simulink model "dinamica_fk"  (Simulink 7.5)
settings: Solver=ode3  StartTime=0.0  StopTime=19.99  FixedStep=0.01  RelTol=1e-3
settings Model: Creator=Granziera  LastModifiedBy=Granziera

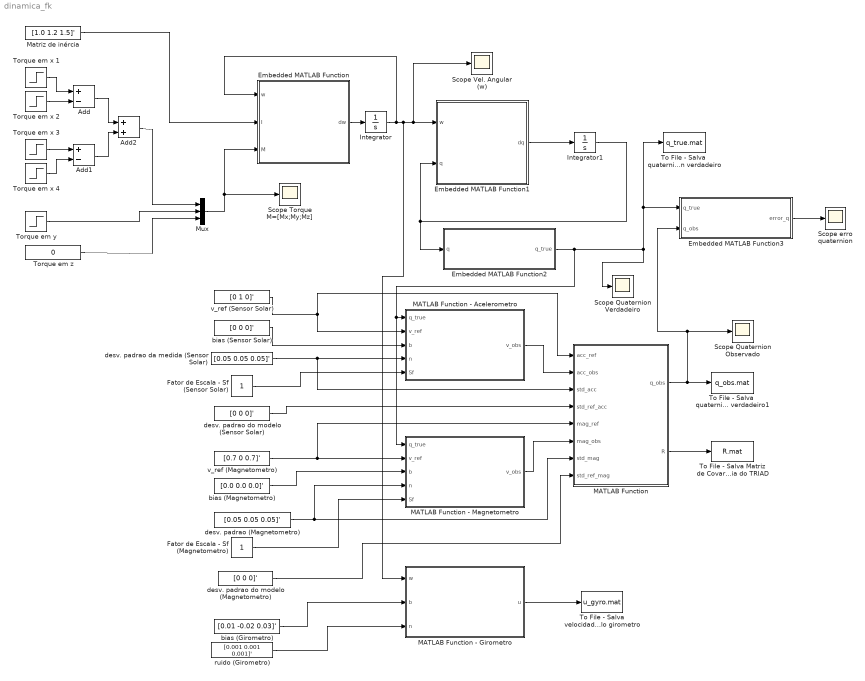
== system dinamica_fk ==
  Add : Sum  Inputs=+-
  Add1 : Sum  Inputs=+-
  Add2 : Sum
  Embedded MATLAB Function : Stateflow chart  TreatAsAtomicUnit=on
  Embedded MATLAB Function1 : Stateflow chart  TreatAsAtomicUnit=on
  Embedded MATLAB Function2 : Stateflow chart  TreatAsAtomicUnit=on
  Embedded MATLAB Function3 : Stateflow chart  TreatAsAtomicUnit=on
  Fator de Escala - Sf (Magnetometro) : Constant
  Fator de Escala - Sf (Sensor Solar) : Constant
  Integrator : Integrator  InitialCondition=[0 0 0]
  Integrator1 : Integrator  InitialCondition=[0 0 0 1]
  MATLAB Function : Stateflow chart  TreatAsAtomicUnit=on
  MATLAB Function - Acelerometro : Stateflow chart  TreatAsAtomicUnit=on
  MATLAB Function - Girometro : Stateflow chart  TreatAsAtomicUnit=on
  MATLAB Function - Magnetometro : Stateflow chart  TreatAsAtomicUnit=on
  Matriz de inércia : Constant  Value=[1.0 1.2 1.5]'
  Mux : Mux  Inputs=3
  Scope Quaternion Observado : Scope
      settings: SaveName=ScopeData3
  Scope Quaternion Verdadeiro : Scope
  Scope Torque M=[Mx;My;Mz] : Scope
      settings: YMin=-0.4  YMax=0.4  SaveName=ScopeData2
  Scope Vel. Angular (w) : Scope
  Scope erro quaternion : Scope
      settings: SaveName=ScopeData5
  To File - Salva  quaternion verdadeiro : ToFile  Filename=q_true.mat  MatrixName=q_true  SaveFormat=Timeseries
  To File - Salva  quaternion verdadeiro1 : ToFile  Filename=q_obs.mat  MatrixName=q_obs  SaveFormat=Timeseries
  To File - Salva Matriz de Covariancia do TRIAD : ToFile  Filename=R.mat  MatrixName=R  SaveFormat=Timeseries
  To File - Salva velocidade angular medida pelo girometro : ToFile  Filename=u_gyro.mat  MatrixName=u_gyro  SaveFormat=Timeseries
  Torque em x 1 : Step  Time=10  After=0.25  SampleTime=0
  Torque em x 2 : Step  Time=11  After=.25  SampleTime=0
  Torque em x 3 : Step  Time=21  After=-.25  SampleTime=0
  Torque em x 4 : Step  Time=22  After=-0.25  SampleTime=0
  "Torque em y " : Step  Time=2  Before=0.1  After=0  SampleTime=0
  Torque em z : Constant  Value=0
  bias (Girometro) : Constant  Value=[0.01 -0.02 0.03]'
  bias (Magnetometro) : Constant  Value=[0.0 0.0 0.0]'
  bias (Sensor Solar) : Constant  Value=[0 0 0]'
  desv. padrao (Magnetometro) : Constant  Value=[0.05 0.05 0.05]'
  desv. padrao da medida (Sensor Solar) : Constant  Value=[0.05 0.05 0.05]'
  desv. padrao do modelo (Magnetometro) : Constant  Value=[0 0 0]'
  desv. padrao do modelo (Sensor Solar) : Constant  Value=[0 0 0]'
  ruido (Girometro) : Constant  Value=[0.001 0.001 0.001]'
  v_ref (Magnetometro) : Constant  Value=[0.7 0 0.7]'
  v_ref (Sensor Solar) : Constant  Value=[0 1 0]'
  wires:
  Matriz de inércia/1 -> Embedded MATLAB Function/2(I)
  Embedded MATLAB Function/1(dw) -> Integrator/1
  Integrator/1 -> Embedded MATLAB Function/1(w), Embedded MATLAB Function1/1(w), Scope Vel. Angular (w)/1, MATLAB Function - Girometro/1(w)
  Mux/1 -> Embedded MATLAB Function/3(M), Scope Torque M=[Mx;My;Mz]/1
  Embedded MATLAB Function1/1(dq) -> Integrator1/1
  Integrator1/1 -> Embedded MATLAB Function1/2(q), Embedded MATLAB Function2/1(q)
  "Torque em y "/1 -> Mux/2
  Torque em z/1 -> Mux/3
  v_ref (Sensor Solar)/1 -> MATLAB Function - Acelerometro/2(v_ref), MATLAB Function/1(acc_ref)
  bias (Sensor Solar)/1 -> MATLAB Function - Acelerometro/3(b)
  desv. padrao da medida (Sensor Solar)/1 -> MATLAB Function - Acelerometro/4(n), MATLAB Function/3(std_acc)
  v_ref (Magnetometro)/1 -> MATLAB Function - Magnetometro/2(v_ref), MATLAB Function/5(mag_ref)
  bias (Magnetometro)/1 -> MATLAB Function - Magnetometro/3(b)
  bias (Girometro)/1 -> MATLAB Function - Girometro/2(b)
  ruido (Girometro)/1 -> MATLAB Function - Girometro/3(n)
  MATLAB Function - Magnetometro/1(v_obs) -> MATLAB Function/6(mag_obs)
  MATLAB Function/2(R) -> To File - Salva Matriz de Covariancia do TRIAD/1
  MATLAB Function - Girometro/1(u) -> To File - Salva velocidade angular medida pelo girometro/1
  desv. padrao (Magnetometro)/1 -> MATLAB Function - Magnetometro/4(n), MATLAB Function/7(std_mag)
  Fator de Escala - Sf (Magnetometro)/1 -> MATLAB Function - Magnetometro/5(Sf)
  Fator de Escala - Sf (Sensor Solar)/1 -> MATLAB Function - Acelerometro/5(Sf)
  desv. padrao do modelo (Sensor Solar)/1 -> MATLAB Function/4(std_ref_acc)
  MATLAB Function/1(q_obs) -> To File - Salva  quaternion verdadeiro1/1, Scope Quaternion Observado/1, Embedded MATLAB Function3/2(q_obs)
  desv. padrao do modelo (Magnetometro)/1 -> MATLAB Function/8(std_ref_mag)
  MATLAB Function - Acelerometro/1(v_obs) -> MATLAB Function/2(acc_obs)
  Embedded MATLAB Function2/1(q_true) -> Scope Quaternion Verdadeiro/1, Embedded MATLAB Function3/1(q_true), To File - Salva  quaternion verdadeiro/1, MATLAB Function - Magnetometro/1(q_true), MATLAB Function - Acelerometro/1(q_true)
  Embedded MATLAB Function3/1(error_q) -> Scope erro quaternion/1
  Torque em x 1/1 -> Add/1
  Torque em x 2/1 -> Add/2
  Torque em x 3/1 -> Add1/1
  Torque em x 4/1 -> Add1/2
  Add1/1 -> Add2/2
  Add/1 -> Add2/1
  Add2/1 -> Mux/1

== matlab function Embedded MATLAB Function1 ==
  data: w input double; dq output double; q input double
function dq = eq_cinematica(w,q)

wx = w(1);
wy = w(2);
wz = w(3);

W = [ 0    wz  -wy  wx;
     -wz   0    wx  wy;
      wy  -wx   0   wz;
     -wx  -wy  -wz  0];

dq = 1/2 * W * q;

== matlab function Embedded MATLAB Function ==
  data: w input double; dw output double; I input double; M input double
function dw = eq_dinamica(w,I,M)

wx = w(1);
wy = w(2);
wz = w(3);

Ix = I(1);
Iy = I(2);
Iz = I(3);

Mx = M(1);
My = M(2);
Mz = M(3);

dx = (Mx - wy*wz*(Iz - Iy)) / Ix;
dy = (My - wx*wz*(Ix - Iz)) / Iy;
dz = (Mz - wx*wy*(Iy - Ix)) / Iz;

dw = [dx dy dz]';

== matlab function MATLAB Function - Magnetometro ==
  data: q_true input double; v_obs output double; v_ref input double; b input double; n input double; Sf input double
function v_obs = Bloco_simula_sensor(q_true,v_ref,b,n,Sf)
%#codegen


% %Operação de transformação de quaternion para Matriz de Rotação
% q2RotMat = [q_true(4).^2 + q_true(1).^2 - q_true(2).^2 - q_true(3).^2 , 2*(q_true(1)*q_true(2) - q_true(4)*q_true(3)) , 2*(q_true(1)*q_true(3) + q_true(4)*q_true(2)) ;...
%     2*(q_true(1)*q_true(2) + q_true(4)*q_true(3)) , q_true(4).^2 - q_true(1).^2 + q_true(2).^2 - q_true(3).^2 , 2*(q_true(2)*q_true(3) - q_true(4)*q_true(1)) ;...
%     2*(q_true(1)*q_true(3) - q_true(4)*q_true(2)), 2*(q_true(2)*q_true(3) + q_true(4)*q_true(1)) , q_true(4).^2 - q_true(1).^2 - q_true(2).^2 + q_true(3).^2];

%Operação de transformação de quaternion para Matriz de Rotação
q2RotMat = [q_true(4).^2 + q_true(1).^2 - q_true(2).^2 - q_true(3).^2 , 2*(q_true(1)*q_true(2) + q_true(4)*q_true(3)) , 2*(q_true(1)*q_true(3) - q_true(4)*q_true(2)) ;...
    2*(q_true(1)*q_true(2) - q_true(4)*q_true(3)) , q_true(4).^2 - q_true(1).^2 + q_true(2).^2 - q_true(3).^2 , 2*(q_true(2)*q_true(3) + q_true(4)*q_true(1)) ;...
    2*(q_true(1)*q_true(3) + q_true(4)*q_true(2)), 2*(q_true(2)*q_true(3) - q_true(4)*q_true(1)) , q_true(4).^2 - q_true(1).^2 - q_true(2).^2 + q_true(3).^2];

%Rotaciona o vetor de observação a partir do vetor de referencia
v_rot = q2RotMat * v_ref;
%Adiciona bias e aplica o fator de escala dos sensores
v_obs = Sf * v_rot + b;
%Adiciona ruido
v_obs = v_obs + n * randn;

== matlab function MATLAB Function - Acelerometro ==
  data: q_true input double; v_obs output double; v_ref input double; b input double; n input double; Sf input double
function v_obs = Bloco_simula_sensor(q_true,v_ref,b,n,Sf)
%#codegen

% %Operação de transformação de quaternion para Matriz de Rotação
% q2RotMat = [q_true(4).^2 + q_true(1).^2 - q_true(2).^2 - q_true(3).^2 , 2*(q_true(1)*q_true(2) - q_true(4)*q_true(3)) , 2*(q_true(1)*q_true(3) + q_true(4)*q_true(2)) ;...
%     2*(q_true(1)*q_true(2) + q_true(4)*q_true(3)) , q_true(4).^2 - q_true(1).^2 + q_true(2).^2 - q_true(3).^2 , 2*(q_true(2)*q_true(3) - q_true(4)*q_true(1)) ;...
%     2*(q_true(1)*q_true(3) - q_true(4)*q_true(2)), 2*(q_true(2)*q_true(3) + q_true(4)*q_true(1)) , q_true(4).^2 - q_true(1).^2 - q_true(2).^2 + q_true(3).^2];

%Operação de transformação de quaternion para Matriz de Rotação
q2RotMat = [q_true(4).^2 + q_true(1).^2 - q_true(2).^2 - q_true(3).^2 , 2*(q_true(1)*q_true(2) + q_true(4)*q_true(3)) , 2*(q_true(1)*q_true(3) - q_true(4)*q_true(2)) ;...
    2*(q_true(1)*q_true(2) - q_true(4)*q_true(3)) , q_true(4).^2 - q_true(1).^2 + q_true(2).^2 - q_true(3).^2 , 2*(q_true(2)*q_true(3) + q_true(4)*q_true(1)) ;...
    2*(q_true(1)*q_true(3) + q_true(4)*q_true(2)), 2*(q_true(2)*q_true(3) - q_true(4)*q_true(1)) , q_true(4).^2 - q_true(1).^2 - q_true(2).^2 + q_true(3).^2];

%Rotaciona o vetor de observação a partir do vetor de referencia
v_rot = q2RotMat * v_ref;
%Adiciona bias e aplica o fator de escala dos sensores
v_obs = Sf * v_rot + b;
%Adiciona ruido
v_obs = v_obs + n * randn;

== matlab function MATLAB Function - Girometro ==
  data: w input double; u output double; b input double; n input double
function u = Bloco_simula_gyro(w,b,n)
%#codegen

%Adiciona bias
u = w + b;
%Adiciona ruido
u = u + n * randn;

== matlab function MATLAB Function ==
  data: acc_ref input double; q_obs output double; acc_obs input double; std_acc input double; std_ref_acc input double; mag_ref input double; mag_obs input double; std_mag input double; R output double; std_ref_mag input double
function [q_obs,R] = TRIAD(acc_ref,acc_obs,std_acc,std_ref_acc,mag_ref,mag_obs,std_mag,std_ref_mag)
%#codegen

%define quaternion de observacao
q_obs= zeros(4,1);

V1 = acc_ref;
W1 = acc_obs;
std_W1 = std_acc';
std_V1 = std_ref_acc';

V2 = mag_ref;
W2 = mag_obs;
std_W2 = std_mag';
std_V2 = std_ref_mag';

%normalizaçao dos vetores

V1 = V1/norm(V1);
W1 = W1/norm(W1);

V2 = V2/norm(V2);
W2 = W2/norm(W2);

%algoritmo TRIAD

M_ref = [ V1 , cross(V1,V2)/norm(cross(V1,V2)) , cross(V1,(cross(V1,V2)))/norm(cross(V1,V2)) ];

M_obs = [ W1 , cross(W1,W2)/norm(cross(W1,W2)) , cross(W1,(cross(W1,W2)))/norm(cross(W1,W2)) ];

A = M_obs * M_ref';

%--------------------------------------------------------------------------
%
%Transformação da Matriz A em quatenion de observacao
%q_obs= [q4,q1,q2,q3];

q_obs(4) = 0.5 * sqrt(trace(A)+1);
q_obs(1) = (A(2,3)-A(3,2))/(4*q_obs(4));
q_obs(2) = (A(3,1)-A(1,3))/(4*q_obs(4));
q_obs(3) = (A(1,2)-A(2,1))/(4*q_obs(4));

%Normalizando o quaternion
q_obs=q_obs/norm(q_obs);

%tira a redundancia do quaternion
if (q_obs(4)<0)
    q_obs=-q_obs;
end

%--------------------------------------------------------------------------



%Calculo da matriz de covariancia

sig1 = sqrt(std_V1.^2 + std_W1.^2);
sig2 = sqrt(std_V2.^2 + std_W2.^2);

% R = sig1.^2 * eye(3) + (1/norm(cross(W1,W2)))^2 * (sig1.^2 * (W1*W2') * (W1*W2' + W2*W1')...
%     + (sig2.^2 - sig1.^2) * W1 * W1');
R = [sig1(1)^2,0,0;0,sig1(2)^2,0;0,0,sig1(3)^2] + (1/norm(cross(W1,W2)))^2 * ([sig1(1)^2,0,0;0,sig1(2)^2,0;0,0,sig1(3)^2] * (W1*W2') * (W1*W2' + W2*W1')...
    + ([sig2(1)^2,0,0;0,sig2(2)^2,0;0,0,sig2(3)^2] - [sig1(1)^2,0,0;0,sig1(2)^2,0;0,0,sig1(3)^2]) * W1 * W1');

== matlab function Embedded MATLAB Function2 ==
  data: q_true output double; q input double
function q_true = tira_redundancia(q)

if(q(4)<0)
    q=-q;
end

q_true=q;

== matlab function Embedded MATLAB Function3 ==
  data: error_q output double; q_true input double; q_obs input double
function error_q  = error_quaternion(q_true,q_obs)
%function [euler_true,euler_obs] = quat2obs(q_true,q_obs)

% %q_true --> euler_true
% psi_true = atan((2*q_true(1)*q_true(2)+2*q_true(4)*q_true(3))/(2*q_true(4)^2+2*q_true(1)^2-1));
% theta_true = asin(-2*q_true(1)*q_true(3)+2*q_true(4)*q_true(1));
% phi_true= atan((2*q_true(2)*q_true(3)+2*q_true(4)*q_true(1))/(2*q_true(4)^2+2*q_true(3)^2-1));
% 
% euler_true = [psi_true,theta_true,phi_true];
% %conversao de radiano para graus
% euler_true = euler_true * 180/pi;
% 
% %q_obs --> euler_obs
% psi_obs = atan((2*q_obs(1)*q_obs(2)+2*q_obs(4)*q_obs(3))/(2*q_obs(4)^2+2*q_obs(1)^2-1));
% theta_obs = asin(-2*q_obs(1)*q_obs(3)+2*q_obs(4)*q_obs(1));
% phi_obs= atan((2*q_obs(2)*q_obs(3)+2*q_obs(4)*q_obs(1))/(2*q_obs(4)^2+2*q_obs(3)^2-1));
% 
% euler_obs = [psi_obs,theta_obs,phi_obs];
% %conversao de radiano para graus
% euler_obs = euler_obs * 180/pi;

%Calcula erro entre q_true e q_obs
if (dot(q_true,q_obs)>0)
 	error_q = q_obs - q_true;
else
 	error_q = -q_obs - q_true;
end
